simulink model "UECU_Speedgoat_threshold"  (R2020b)
settings: Solver=FixedStepDiscrete  StartTime=0.0  StopTime=inf  RelTol=1e-3  EnableMultiTasking=on
PreLoadFcn:
  | Ts=1e-3;
libraries: devices x5, simulink x2
settings Model: SimulationMode=external  Creator=Matthew  LastModifiedBy=Speedgoat-5
settings SolverCC: ConcurrentTasks=on  PositivePriorityOrder=on
settings DataIOCC: LimitDataPoints=on  SaveFormat=Array  SignalLoggingSaveFormat=ModelDataLogs  ReturnWorkspaceOutputs=off
settings OptimizationCC: BlockReduction=off  OptimizeBlockIOStorage=off  BufferReuse=off  ExpressionFolding=off  ExpressionDepthLimit=2147483647  LocalBlockOutputs=off  InitFltsAndDblsToZero=on
settings DebuggingCC: SaveWithParameterizedLinksMsg=none  UnderspecifiedInitializationDetection=Classic  MergeDetectMultiDrivingBlocksExec=none  SignalResolutionControl=TryResolveAllWithWarning  SolverPrmCheckMsg=warning  InheritedTsInSrcMsg=none  FcnCallInpInsideContextMsg=warning  StateNameClashWarn=warning  SFUnexpectedBacktrackingDiag=warning  SFNoUnconditionalDefaultTransitionDiag=warning  SFExecutionAtInitializationDiag=none  ArithmeticOperatorsInVariantConditions=warning
settings HardwareCC: ProdBitPerLong=64  ProdLongLongMode=on  ProdHWDeviceType=Intel->x86-64 (Linux 64)  TargetHWDeviceType=32-bit Generic
settings ModelReferenceCC: PropagateSignalLabelsOutOfModel=off
settings SFSimCC: SimUseLocalCustomCode=off  CustomCodeUndefinedFunction=UseInterfaceOnly
settings RTWCC: Description=Simulink Real-Time  SystemTargetFile=slrealtime.tlc  TemplateMakefile=slrealtime_default_tmf  RTWUseLocalCustomCode=off  Toolchain=Simulink Real-Time Toolchain  BuildConfiguration=Faster Runs  CodeExecutionProfiling=on  TargetLang=C++
settings CodeAppCC: StateflowObjectComments=on
settings ConfigComp: CovMetricSettings=dw  CovSaveCumulativeToWorkspaceVar=on  CovSaveSingleToWorkspaceVar=on  CovExternalEMLEnable=off

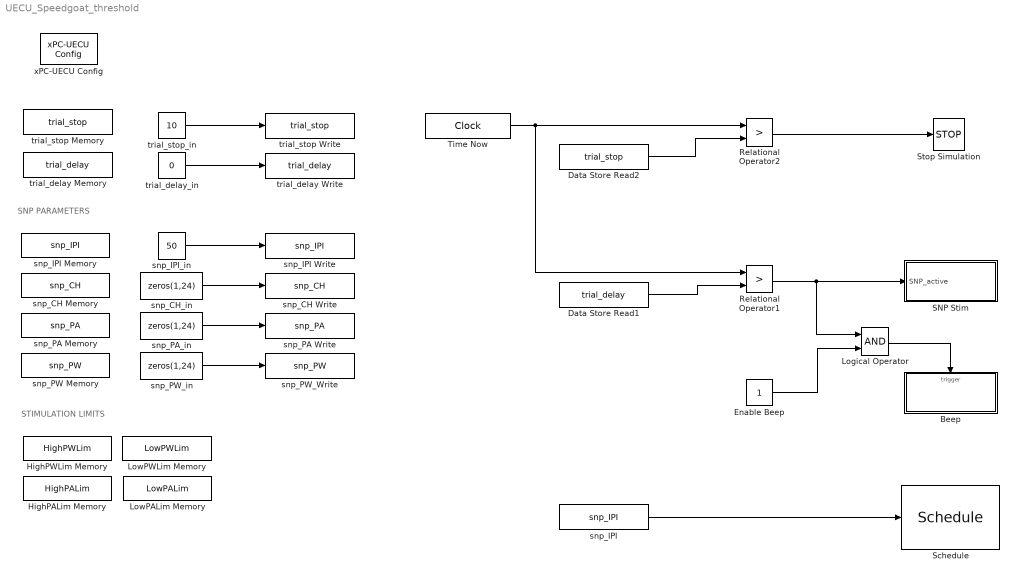
== system UECU_Speedgoat_threshold ==
  note: STIMULATION LIMITS
  note: SNP PARAMETERS
  Beep : Subsystem  TreatAsAtomicUnit=on
  Data Store Read1 : DataStoreRead  DataStoreName=trial_delay
  Data Store Read2 : DataStoreRead  DataStoreName=trial_stop  SampleTime=Ts
  Enable Beep : Constant  OutDataTypeStr=boolean  SampleTime=Ts
  HighPALim Memory : DataStoreMemory  DataStoreName=HighPALim  ReadBeforeWriteMsg=warning  WriteAfterWriteMsg=warning  WriteAfterReadMsg=warning  InitialValue=5.6  ShowAdditionalParam=off
  HighPWLim Memory : DataStoreMemory  DataStoreName=HighPWLim  ReadBeforeWriteMsg=warning  WriteAfterWriteMsg=warning  WriteAfterReadMsg=warning  InitialValue=255  ShowAdditionalParam=off
  Logical Operator : Logic  AllPortsSameDT=off  OutDataTypeStr=boolean
  LowPALim Memory : DataStoreMemory  DataStoreName=LowPALim  ReadBeforeWriteMsg=warning  WriteAfterWriteMsg=warning  WriteAfterReadMsg=warning  ShowAdditionalParam=off
  LowPWLim Memory : DataStoreMemory  DataStoreName=LowPWLim  ReadBeforeWriteMsg=warning  WriteAfterWriteMsg=warning  WriteAfterReadMsg=warning  ShowAdditionalParam=off
  Relational Operator1 : RelationalOperator  Operator=>  OutDataTypeStr=boolean  SampleTime=Ts  RndMeth=Nearest
  Relational Operator2 : RelationalOperator  Operator=>  OutDataTypeStr=boolean  SampleTime=Ts  RndMeth=Nearest
  SNP Stim : Subsystem  TreatAsAtomicUnit=on
  Schedule : devices/Schedule  sched=schedule1  stype=Variable  period=80  t=Ts
      settings: SourceProductName=UECU
  Stop Simulation : Stop
  Time Now : DigitalClock  SampleTime=Ts
  snp_CH Memory : DataStoreMemory  DataStoreName=snp_CH  ReadBeforeWriteMsg=warning  WriteAfterWriteMsg=warning  WriteAfterReadMsg=warning  InitialValue=zeros(1,24)  ShowAdditionalParam=off  OutDataTypeStr=boolean
  snp_CH Write : DataStoreWrite  DataStoreName=snp_CH  SampleTime=Ts
  snp_CH_in : Constant  Value=zeros(1,24)  OutDataTypeStr=boolean  SampleTime=Ts
  snp_IPI : DataStoreRead  DataStoreName=snp_IPI  SampleTime=Ts
  snp_IPI Memory : DataStoreMemory  DataStoreName=snp_IPI  ReadBeforeWriteMsg=warning  WriteAfterWriteMsg=warning  WriteAfterReadMsg=warning  ShowAdditionalParam=off  OutDataTypeStr=uint16
  snp_IPI Write : DataStoreWrite  DataStoreName=snp_IPI  SampleTime=Ts
  snp_IPI_in : Constant  Value=50  OutDataTypeStr=uint16  SampleTime=Ts
  snp_PA Memory : DataStoreMemory  DataStoreName=snp_PA  ReadBeforeWriteMsg=warning  WriteAfterWriteMsg=warning  WriteAfterReadMsg=warning  InitialValue=zeros(1,24)  ShowAdditionalParam=off  OutDataTypeStr=double
  snp_PA Write : DataStoreWrite  DataStoreName=snp_PA  SampleTime=Ts
  snp_PA_in : Constant  Value=zeros(1,24)  OutDataTypeStr=double  SampleTime=Ts
  snp_PW Memory : DataStoreMemory  DataStoreName=snp_PW  ReadBeforeWriteMsg=warning  WriteAfterWriteMsg=warning  WriteAfterReadMsg=warning  InitialValue=zeros(1,24)  ShowAdditionalParam=off  OutDataTypeStr=uint8
  snp_PW_Write : DataStoreWrite  DataStoreName=snp_PW  SampleTime=Ts
  snp_PW_in : Constant  Value=zeros(1,24)  OutDataTypeStr=uint8  SampleTime=Ts
  trial_delay Memory : DataStoreMemory  DataStoreName=trial_delay  ReadBeforeWriteMsg=warning  WriteAfterWriteMsg=warning  WriteAfterReadMsg=warning  ShowAdditionalParam=off
  trial_delay Write : DataStoreWrite  DataStoreName=trial_delay
  trial_delay_in : Constant  Value=0  SampleTime=Ts
  trial_stop Memory : DataStoreMemory  DataStoreName=trial_stop  ReadBeforeWriteMsg=warning  WriteAfterWriteMsg=warning  WriteAfterReadMsg=warning  ShowAdditionalParam=off
  trial_stop Write : DataStoreWrite  DataStoreName=trial_stop
  trial_stop_in : Constant  Value=10  SampleTime=Ts
  xPC-UECU Config : devices/xPC Functions/xPC-UECU Config  port=COM2  baud=115200  flowctrl=on  addr=128
      settings: SourceProductName=UECU
  wires:
  snp_CH_in/1 -> snp_CH Write/1
  snp_PA_in/1 -> snp_PA Write/1
  snp_PW_in/1 -> snp_PW_Write/1
  snp_IPI_in/1 -> snp_IPI Write/1
  snp_IPI/1 -> Schedule/1
  trial_delay_in/1 -> trial_delay Write/1
  trial_stop_in/1 -> trial_stop Write/1
  Data Store Read2/1 -> Relational Operator2/2
  Time Now/1 -> Relational Operator2/1, Relational Operator1/1
  Relational Operator2/1 -> Stop Simulation/1
  Data Store Read1/1 -> Relational Operator1/2
  Relational Operator1/1 -> Logical Operator/1, SNP Stim/1(SNP_active)
  Logical Operator/1 -> Beep/Trigger
  Enable Beep/1 -> Logical Operator/2

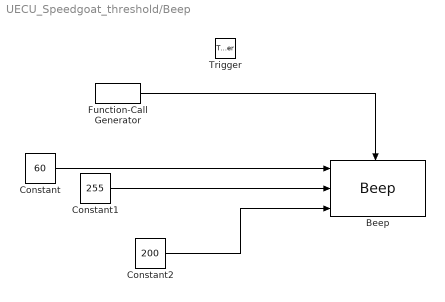
== system UECU_Speedgoat_threshold/Beep ==
  Trigger : TriggerPort  VariantControl=(inherit)
  Beep : devices/Sound/Beep  addr=0  sm=11
      settings: SourceProductName=UECU
  Constant : Constant  Value=60  OutDataTypeStr=uint8  SampleTime=-1
  Constant1 : Constant  Value=255  OutDataTypeStr=uint8  SampleTime=-1
  Constant2 : Constant  Value=200  OutDataTypeStr=uint16  SampleTime=-1
  Function-Call Generator : simulink/Ports & Subsystems/Function-Call Generator  sample_time=-1  numberOfIterations=1  DisallowWideOutput=off
  wires:
  Function-Call Generator/1 -> Beep/Trigger
  Constant/1 -> Beep/1
  Constant1/1 -> Beep/2
  Constant2/1 -> Beep/3

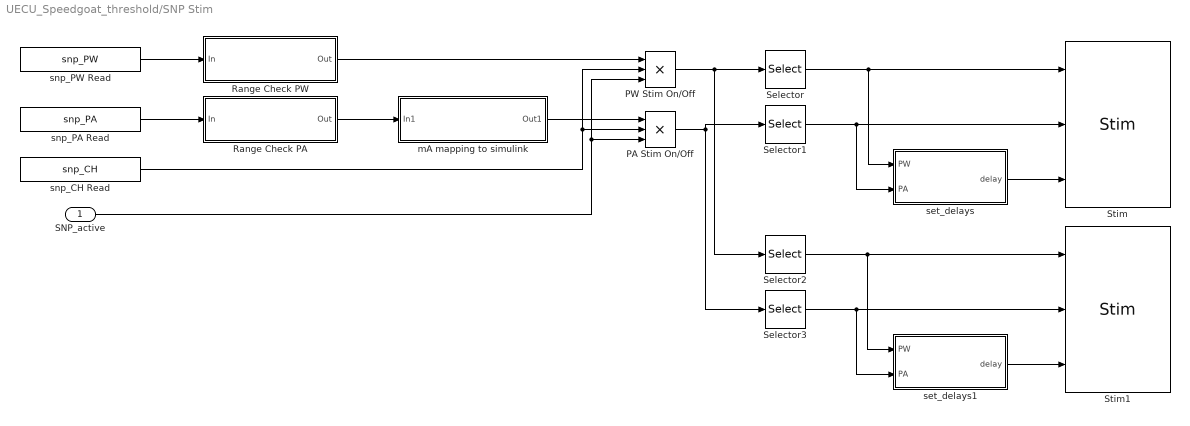
== system UECU_Speedgoat_threshold/SNP Stim ==
  SNP_active : Inport  OutDataTypeStr=boolean
  PA Stim On/Off : Product  Inputs=***  OutDataTypeStr=uint8  SampleTime=Ts
  PW Stim On/Off : Product  Inputs=***  OutDataTypeStr=uint8  SampleTime=Ts
  Range Check PA : Subsystem
  Range Check PW : Subsystem
  Selector : Selector  IndexMode=Zero-based  InputPortWidth=24  IndexOptions=Index vector (dialog)  Indices=[0:11]  OutputSizes=1
  Selector1 : Selector  IndexMode=Zero-based  InputPortWidth=24  IndexOptions=Index vector (dialog)  Indices=[0:11]  OutputSizes=1
  Selector2 : Selector  IndexMode=Zero-based  InputPortWidth=24  IndexOptions=Index vector (dialog)  Indices=[12:23]  OutputSizes=1
  Selector3 : Selector  IndexMode=Zero-based  InputPortWidth=24  IndexOptions=Index vector (dialog)  Indices=[12:23]  OutputSizes=1
  Stim : devices/Stim  addr=1  port=0  chan=[0:11]  dselect=Input  delays=5*ones(1,12)  autosched=Manual  sched=schedule1  pri=100  period=Ts
      settings: SourceProductName=UECU
  Stim1 : devices/Stim  addr=2  port=0  chan=[0:11]  dselect=Input  delays=5*ones(1,12)  autosched=Manual  sched=schedule1  pri=100  period=Ts
      settings: SourceProductName=UECU
  mA mapping to simulink : Subsystem
  set_delays : MATLAB Function  TreatAsAtomicUnit=on
  set_delays1 : MATLAB Function  TreatAsAtomicUnit=on
  snp_CH Read : DataStoreRead  DataStoreName=snp_CH  SampleTime=Ts
  snp_PA Read : DataStoreRead  DataStoreName=snp_PA  SampleTime=Ts
  snp_PW Read : DataStoreRead  DataStoreName=snp_PW  SampleTime=Ts
  wires:
  snp_PW Read/1 -> Range Check PW/1(In)
  snp_PA Read/1 -> Range Check PA/1(In)
  Selector1/1 -> Stim/2, set_delays/2(PA)
  Range Check PA/1(Out) -> mA mapping to simulink/1(In1)
  Selector/1 -> set_delays/1(PW), Stim/1
  Selector2/1 -> set_delays1/1(PW), Stim1/1
  Selector3/1 -> Stim1/2, set_delays1/2(PA)
  SNP_active/1 -> PA Stim On/Off/3, PW Stim On/Off/3
  Range Check PW/1(Out) -> PW Stim On/Off/1
  mA mapping to simulink/1(Out1) -> PA Stim On/Off/1
  snp_CH Read/1 -> PA Stim On/Off/2, PW Stim On/Off/2
  PW Stim On/Off/1 -> Selector2/1, Selector/1
  PA Stim On/Off/1 -> Selector3/1, Selector1/1
  set_delays/1(delay) -> Stim/3
  set_delays1/1(delay) -> Stim1/3

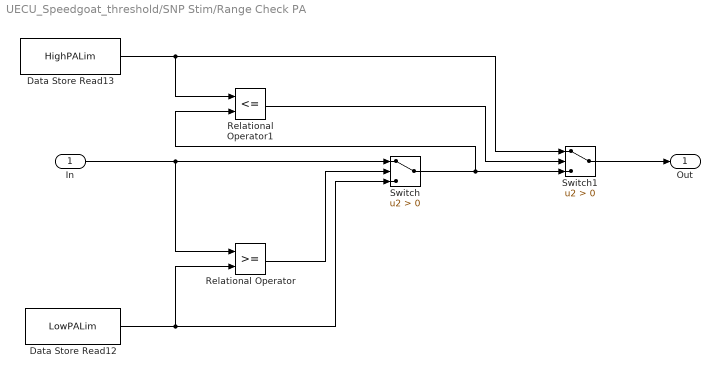
== system UECU_Speedgoat_threshold/SNP Stim/Range Check PA ==
  In : Inport  OutDataTypeStr=double
  Data Store Read12 : DataStoreRead  DataStoreName=LowPALim  SampleTime=Ts
  Data Store Read13 : DataStoreRead  DataStoreName=HighPALim  SampleTime=Ts
  Relational Operator : RelationalOperator  OutDataTypeStr=boolean  SampleTime=Ts  RndMeth=Nearest
  Relational Operator1 : RelationalOperator  Operator=<=  OutDataTypeStr=boolean  SampleTime=Ts  RndMeth=Nearest
  Switch : Switch  Criteria=u2 > Threshold  SampleTime=Ts
  Switch1 : Switch  Criteria=u2 > Threshold  SampleTime=Ts
  Out : Outport  OutDataTypeStr=double
  wires:
  Relational Operator/1 -> Switch/2
  Data Store Read13/1 -> Relational Operator1/1, Switch1/1
  Switch/1 -> Relational Operator1/2, Switch1/3
  Relational Operator1/1 -> Switch1/2
  In/1 -> Relational Operator/1, Switch/1
  Data Store Read12/1 -> Relational Operator/2, Switch/3
  Switch1/1 -> Out/1

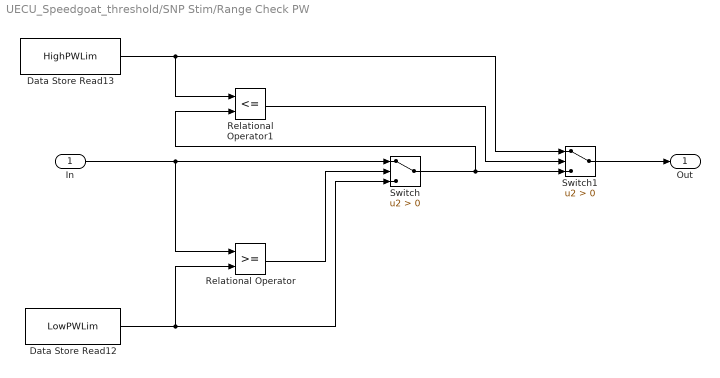
== system UECU_Speedgoat_threshold/SNP Stim/Range Check PW ==
  In : Inport  OutDataTypeStr=uint8
  Data Store Read12 : DataStoreRead  DataStoreName=LowPWLim  SampleTime=Ts
  Data Store Read13 : DataStoreRead  DataStoreName=HighPWLim  SampleTime=Ts
  Relational Operator : RelationalOperator  OutDataTypeStr=boolean  SampleTime=Ts  RndMeth=Nearest
  Relational Operator1 : RelationalOperator  Operator=<=  OutDataTypeStr=boolean  SampleTime=Ts  RndMeth=Nearest
  Switch : Switch  Criteria=u2 > Threshold  SampleTime=Ts
  Switch1 : Switch  Criteria=u2 > Threshold  SampleTime=Ts
  Out : Outport  OutDataTypeStr=uint8
  wires:
  Relational Operator/1 -> Switch/2
  Data Store Read13/1 -> Relational Operator1/1, Switch1/1
  Switch/1 -> Relational Operator1/2, Switch1/3
  Relational Operator1/1 -> Switch1/2
  In/1 -> Relational Operator/1, Switch/1
  Data Store Read12/1 -> Relational Operator/2, Switch/3
  Switch1/1 -> Out/1

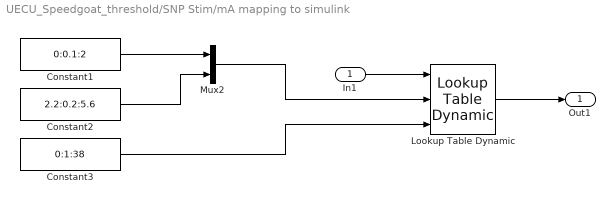
== system UECU_Speedgoat_threshold/SNP Stim/mA mapping to simulink ==
  In1 : Inport  OutDataTypeStr=double  PortDimensions=24
  Constant1 : Constant  Value=0:0.1:2  OutDataTypeStr=double
  Constant2 : Constant  Value=2.2:0.2:5.6  OutDataTypeStr=double
  Constant3 : Constant  Value=0:1:38  OutDataTypeStr=uint8
  Lookup Table Dynamic : simulink/Lookup Tables/Lookup Table Dynamic  LookUpMeth=Interpolation-Use End Values  OutDataType=fixdt('uint8')  OutScaling=[]  OutputDataTypeScalingMode=Specify via dialog  OutDataTypeStr=fixdt('uint8')  DoSatur=off
  Mux2 : Mux  Inputs=2
  Out1 : Outport  OutDataTypeStr=uint8
  wires:
  Constant1/1 -> Mux2/1
  Constant2/1 -> Mux2/2
  Mux2/1 -> Lookup Table Dynamic/2
  Constant3/1 -> Lookup Table Dynamic/3
  In1/1 -> Lookup Table Dynamic/1
  Lookup Table Dynamic/1 -> Out1/1

== matlab function UECU_Speedgoat_threshold/SNP Stim/set_delays ==
  data: PW input; delay output; PA input
function delay = set_delays(PW, PA)

PWA = PW.*PA; % figure out which channels have stim
L = length(PWA(PWA~=0)); % find the total number of channels with stim
d = uint8(1:L); % set the delay vector based on the number of channels with stim
PWA(PWA~=0) = d;
delay=uint16(PWA);

== matlab function UECU_Speedgoat_threshold/SNP Stim/set_delays1 ==
  data: PW input; delay output; PA input
function delay = set_delays(PW, PA)

PWA = PW.*PA; % figure out which channels have stim
L = length(PWA(PWA~=0)); % find the total number of channels with stim
d = uint8(1:L); % set the delay vector based on the number of channels with stim
PWA(PWA~=0) = d;
delay=uint16(PWA);
